simulink model "SistemaNoLinealYMascara"  (R2019a)
settings: Solver=ode8  StartTime=0  StopTime=10e-35  RelTol=1e-3
values from neighbouring files (symbols this model uses):
  C = 10e-6    (= 1e-05)    [Grafico1.m]
  E = 10    [Grafico1.m]
  L = 4.9e-3    (= 0.0049)    [Grafico1.m]
  R = 220    [Grafico1.m]
  U = 0.5    [Grafico1.m]
settings Model: Creator=franc  LastModifiedBy=franc

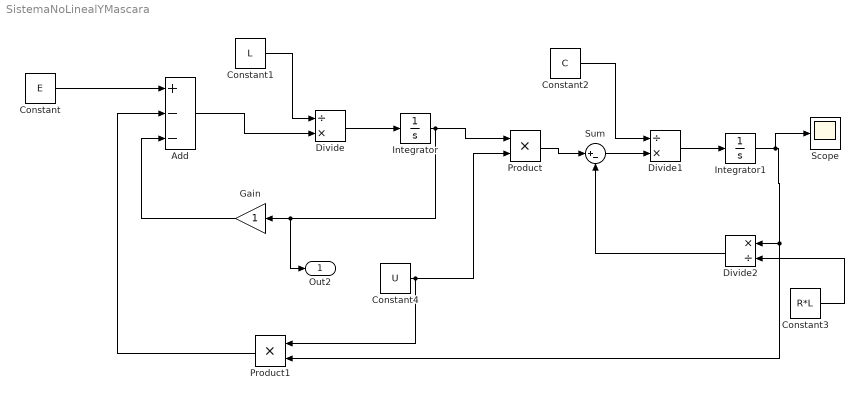
== system SistemaNoLinealYMascara ==
  Add : Sum  Inputs=+--
  Constant : Constant  Value=E
  Constant1 : Constant  Value=L
  Constant2 : Constant  Value=C
  Constant3 : Constant  Value=R*L
  Constant4 : Constant  Value=U
  Divide : Product  Inputs=/*
  Divide1 : Product  Inputs=/*
  Divide2 : Product  Inputs=*/
  Gain : Gain
  Integrator : Integrator
  Integrator1 : Integrator
  Product : Product
  Product1 : Product
  Scope : Scope
  Sum : Sum  Inputs=|+-
  Out2 : Outport
  wires:
  Constant/1 -> Add/1
  Constant1/1 -> Divide/1
  Add/1 -> Divide/2
  Divide/1 -> Integrator/1
  Integrator/1 -> Out2/1, Gain/1, Product/1
  Gain/1 -> Add/3
  Product/1 -> Sum/1
  Sum/1 -> Divide1/2
  Constant2/1 -> Divide1/1
  Divide1/1 -> Integrator1/1
  Integrator1/1 -> Scope/1, Product1/2, Divide2/1
  Constant3/1 -> Divide2/2
  Divide2/1 -> Sum/2
  Product1/1 -> Add/2
  Constant4/1 -> Product1/1, Product/2
